simulink library "xpcmeasurementcomputinglib"  (Simulink 6.0)
settings: Solver=ode45  SolverMode=SingleTasking  StartTime=0.0  StopTime=10.0  RelTol=1e-3
values from neighbouring files (symbols this model uses):
  channels = round(channels)    [mbwaudpmc.m]
undefined symbols (not defined in the file or in its folder): madcbciodas, madcbpcidas, madcbpcidas1600, mctr05checks, mdacbisa, mdacbpcidas, mdacbpcidas1600, mdacbpcidda0x12, mdiocbpcipdisox, menccbcioquadcount, misa8255, mpci8255, mtccb
libraries: xpcmeasurementcomputinglib x18
(part 1 of 4)
settings Model: Creator=adowd  LastModifiedBy=gweast
settings DataIOCC: SignalLoggingName=logsOut
settings OptimizationCC: BooleanDataType=off
settings DebuggingCC: CheckExecutionContextPreStartOutputMsg=on  CheckExecutionContextRuntimeOutputMsg=on  SolverPrmCheckMsg=none
settings HardwareCC: TargetUnknown=on
settings GRTTargetCC: UtilityFuncGeneration=Automatic  LifeSpan=inf
settings SFSimCC: SFSimApplyToAllLibs=on  SFSimBuildMode=Incremental

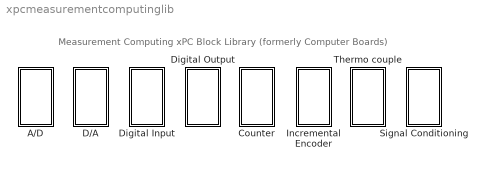
== system xpcmeasurementcomputinglib ==
  note: Measurement Computing xPC Block Library
      | (formerly Computer Boards)
  A/D : Subsystem  EnableExecutionContextPropagation=on
  Counter : Subsystem  EnableExecutionContextPropagation=on
  D/A : Subsystem  EnableExecutionContextPropagation=on
  Digital Input : Subsystem  EnableExecutionContextPropagation=on
  Digital Output : Subsystem  EnableExecutionContextPropagation=on
  Incremental Encoder : Subsystem  EnableExecutionContextPropagation=on
  Signal Conditioning : Subsystem  EnableExecutionContextPropagation=on
  Thermo couple : Subsystem  EnableExecutionContextPropagation=on

== system xpcmeasurementcomputinglib/A/D ==
  "CIO-DAS16 330 " : S-Function  InitFcn=madcbciodas(1);  FunctionName=adcbciodas  Parameters="channel, range, gain, offset, control, mux, sampletime, baseaddress,  boardType"  mask(adcbpcidas){channel=1, range=+-10V, mux=Single-ended (16 channels), sampletime=0.001, baseaddress=0x300}
      mask prompts: channel "Number of channels:"; range "Range vector:"; mux "Input coupling:"; sampletime "Sample time:"; baseaddress "Base address (i.e. 0xd000):"
      mask help:
      | CIO-DAS16/300
      | ComputerBoards
      | Analog Input
      mask init:
      | baseaddress=hex2dec(baseaddress(3:end));
      | boardType=4;gain=0;offset=0;control=0;
      | [gain, offset, control]=madcbciodas(2, channel, range, mux, baseaddress, boardType);
      mask Help: helpview(fullfile(docroot, 'mapfiles', 'xpc.map'), 'ComputerBoards_CIO-DAS16-330_AD')
      mask StyleString: edit,popup(+-10V|+-5V|+-2.5V|+-1.25V|+-0.625V|0-10V|0-5V|0-2.5V|0-1.25V),popup(Single-ended (16 channels)|differential (8 channels)),edit,edit
      mask Display: disp('CIO-DAS16/330\nComputerBoards\nAnalog Input');port_label('output',1,'1');
  "CIO-DAS16 JR " : S-Function  InitFcn=madcbciodas(1);  FunctionName=adcbciodas  Parameters="channel, range, gain, offset, control, mux, sampletime, baseaddress,  boardType"  mask(adcbpcidas){channel=1, range=+-10V, mux=Single-ended (16 channels), sampletime=0.001, baseaddress=0x300}
      mask prompts: channel "Number of channels:"; range "Range vector:"; mux "Input coupling:"; sampletime "Sample time:"; baseaddress "Base address (i.e. 0xd000):"
      mask help:
      | CIO-DAS16/JR
      | ComputerBoards
      | Analog Input
      mask init:
      | baseaddress=hex2dec(baseaddress(3:end));
      | boardType=1;gain=0;offset=0;control=0;
      | [gain, offset, control]=madcbciodas(2, channel, range, mux, baseaddress, boardType);
      mask Help: helpview(fullfile(docroot, 'mapfiles', 'xpc.map'), 'ComputerBoards_CIO-DAS16-JR_AD')
      mask StyleString: edit,popup(+-10V|+-5V|+-2.5V|+-1.25V|+-0.625V|0-10V|0-5V|0-2.5V|0-1.25V),popup(Single-ended (16 channels)|differential (8 channels)),edit,edit
      mask Display: disp('CIO-DAS16/JR\nComputerBoards\nAnalog Input');port_label('output',1,'1');
  "CIO-DAS1601 12 " : S-Function  InitFcn=madcbciodas(1);  FunctionName=adcbciodas  Parameters="channel, range, gain, offset, control, mux, sampletime, baseaddress,  boardType"  mask(adcbpcidas){channel=1, range=+-10V, mux=Single-ended (16 channels), sampletime=0.001, baseaddress=0x300}
      mask prompts: channel "Number of channels:"; range "Range vector:"; mux "Input coupling:"; sampletime "Sample time:"; baseaddress "Base address (i.e. 0xd000):"
      mask help:
      | CIO-DAS1601/12
      | ComputerBoards
      | Analog Input
      mask init:
      | baseaddress=hex2dec(baseaddress(3:end));
      | boardType=2;gain=0;offset=0;control=0;
      | [gain, offset, control]=madcbciodas(2, channel, range, mux, baseaddress, boardType);
      mask Help: helpview(fullfile(docroot, 'mapfiles', 'xpc.map'), 'ComputerBoards_CIO-DAS1601-12_AD')
      mask StyleString: edit,popup(+-10V|+-1V|+-0.1V|+-0.01V|0-10V|0-1V|0-0.1V|0-0.01V),popup(Single-ended (16 channels)|Differential (8 channels)),edit,edit
      mask Display: disp('CIO-DAS1601/12\nComputerBoards\nAnalog Input');port_label('output',1,'1');
  "CIO-DAS1602 12 " : S-Function  InitFcn=madcbciodas(1);  FunctionName=adcbciodas  Parameters="channel, range, gain, offset, control, mux, sampletime, baseaddress,  boardType"  mask(adcbpcidas){channel=1, range=+-10V, mux=Single-ended (16 channels), sampletime=0.001, baseaddress=0x300}
      mask prompts: channel "Number of channels:"; range "Range vector:"; mux "Input coupling:"; sampletime "Sample time:"; baseaddress "Base address (i.e. 0xd000):"
      mask help:
      | CIO-DAS1602/12
      | ComputerBoards
      | Analog Input
      mask init:
      | baseaddress=hex2dec(baseaddress(3:end));
      | boardType=3;gain=0;offset=0;control=0;
      | [gain, offset, control]=madcbciodas(2, channel, range, mux, baseaddress, boardType);
      mask Help: helpview(fullfile(docroot, 'mapfiles', 'xpc.map'), 'ComputerBoards_CIO-DAS1602-12_AD')
      mask StyleString: edit,popup(+-10V|+-5V|+-2.5V|+-1.25V|0-10V|0-5V|0-2.5V|0-1.25V),popup(Single-ended (16 channels)|Differential (8 channels)),edit,edit
      mask Display: disp('CIO-DAS1602/12\nComputerBoards\nAnalog Input');port_label('output',1,'1');
  "CIO-DAS1602 16 " : S-Function  InitFcn=madcbciodas(1);  FunctionName=adcbciodas  Parameters="channel, range, gain, offset, control, mux, sampletime, baseaddress,  boardType"  mask(adcbpcidas){channel=1, range=+-10V, mux=Single-ended (16 channels), sampletime=0.001, baseaddress=0x300}
      mask prompts: channel "Number of channels:"; range "Range vector:"; mux "Input coupling:"; sampletime "Sample time:"; baseaddress "Base address (i.e. 0xd000):"
      mask help:
      | CIO-DAS1602/16
      | ComputerBoards
      | Analog Input
      mask init:
      | baseaddress=hex2dec(baseaddress(3:end));
      | boardType=7;gain=0;offset=0;control=0;
      | [gain, offset, control]=madcbciodas(2, channel, range, mux, baseaddress, boardType);
      mask Help: helpview(fullfile(docroot, 'mapfiles', 'xpc.map'), 'ComputerBoards_CIO-DAS1602-16_AD')
      mask StyleString: edit,popup(+-10V|+-5V|+-2.5V|+-1.25V|+-0.625V|0-10V|0-5V|0-2.5V|0-1.25V),popup(Single-ended (16 channels)|differential (8 channels)),edit,edit
      mask Display: disp('CIO-DAS1602/16\nComputerBoards\nAnalog Input');port_label('output',1,'1');
  "CIO-DAS16JR 16 " : S-Function  InitFcn=madcbciodas(1);  FunctionName=adcbciodas  Parameters="channel, range, gain, offset, control, mux, sampletime, baseaddress,  boardType"  mask(adcbpcidas){channel=1, range=+-10V, mux=Single-ended (16 channels), sampletime=0.001, baseaddress=0x300}
      mask prompts: channel "Number of channels:"; range "Range vector:"; mux "Input coupling:"; sampletime "Sample time:"; baseaddress "Base address (i.e. 0xd000):"
      mask help:
      | CIO-DAS16JR/16
      | ComputerBoards
      | Analog Input
      mask init:
      | baseaddress=hex2dec(baseaddress(3:end));
      | boardType=6;gain=0;offset=0;control=0;
      | [gain, offset, control]=madcbciodas(2, channel, range, mux, baseaddress, boardType);
      mask Help: helpview(fullfile(docroot, 'mapfiles', 'xpc.map'), 'ComputerBoards_CIO-DAS16JR-16_AD')
      mask StyleString: edit,popup(+-10V|+-5V|+-2.5V|+-1.25V|+-0.625V|0-10V|0-5V|0-2.5V|0-1.25V),popup(Single-ended (16 channels)|differential (8 channels)),edit,edit
      mask Display: disp('CIO-DAS16JR/16\nComputerBoards\nAnalog Input');port_label('output',1,'1');
  "CIO-DAS16JR EXP " : Subsystem  EnableExecutionContextPropagation=on  mask(Analog Input Module){channels=[], gain=[], admux=0, range=+-10V, sampletime=0.001, baseaddress=0x300}
      mask prompts: channels "EXP channel vector:"; gain "EXP gain vector:"; admux "A/D board channel:"; range "A/D board range:"; sampletime "Sample time:"; baseaddress "Base address (i.e. 0xd000):"
      mask help:
      | Computer Boards
      | CIO-DAS16/Jr with EXP
      | Analog Input
      mask init:
      | baseaddress=hex2dec(baseaddress(3:end));
      mask Help: helpview(fullfile(docroot, 'mapfiles', 'xpc.map'), 'ComputerBoards_CIO-DAS16JR-EXP_AD')
      mask StyleString: edit,edit,popup(0|1|2|3|4|5|6|7|8|9|10|11|12|13|14|15),popup(+-10V|+-5V|+-2.5V|+-1.25V|+-0.625V|0-10V|0-5V|0-2.5V|0-1.25V),edit,edit
      mask Display: disp('CIO-DAS16/Jr EXP\nComputerBoards\nAnalog Input')
  "PC104-DAS16JR 12 " : S-Function  InitFcn=madcbciodas(1);  FunctionName=adcbciodas  Parameters="channel, range, gain, offset, control, mux, sampletime, baseaddress,  boardType"  mask(adcbpcidas){channel=1, range=+-10V, mux=Single-ended (16 channels), sampletime=0.001, baseaddress=0x300}
      mask prompts: channel "Number of channels:"; range "Range vector:"; mux "Input coupling:"; sampletime "Sample time:"; baseaddress "Base address (i.e. 0xd000):"
      mask help:
      | PC104-DAS16JR/12
      | ComputerBoards
      | Analog Input
      mask init:
      | baseaddress=hex2dec(baseaddress(3:end));
      | boardType=5;gain=0;offset=0;control=0;
      | [gain, offset, control]=madcbciodas(2, channel, range, mux, baseaddress, boardType);
      mask Help: helpview(fullfile(docroot, 'mapfiles', 'xpc.map'), 'ComputerBoards_PC104-DAS16JR-12_AD')
      mask StyleString: edit,popup(+-10V|+-5V|+-2.5V|+-1.25V|+-0.625V|0-10V|0-5V|0-2.5V|0-1.25V),popup(Single-ended (16 channels)|differential (8 channels)),edit,edit
      mask Display: disp('PC104-DAS16JR/12\nComputerBoards\nAnalog Input');port_label('output',1,'1');
  "PC104-DAS16JR 16 " : S-Function  InitFcn=madcbciodas(1);  FunctionName=adcbciodas  Parameters="channel, range, gain, offset, control, mux, sampletime, baseaddress,  boardType"  mask(adcbpcidas){channel=1, range=+-10V, mux=Single-ended (16 channels), sampletime=0.001, baseaddress=0x300}
      mask prompts: channel "Number of channels:"; range "Range vector:"; mux "Input coupling:"; sampletime "Sample time:"; baseaddress "Base address (i.e. 0xd000):"
      mask help:
      | PC104-DAS16JR/16
      | ComputerBoards
      | Analog Input
      mask init:
      | baseaddress=hex2dec(baseaddress(3:end));
      | boardType=8;gain=0;offset=0;control=0;
      | [gain, offset, control]=madcbciodas(2, channel, range, mux, baseaddress, boardType);
      mask Help: helpview(fullfile(docroot, 'mapfiles', 'xpc.map'), 'ComputerBoards_PC104-DAS16JR-16_AD')
      mask StyleString: edit,popup(+-10V|+-5V|+-2.5V|+-1.25V|+-0.625V|0-10V|0-5V|0-2.5V|0-1.25V),popup(Single-ended (16 channels)|differential (8 channels)),edit,edit
      mask Display: disp('PC104-DAS16JR/16\nComputerBoards\nAnalog Input');port_label('output',1,'1');
  "PCI-DAS1200 " : S-Function  InitFcn=madcbpcidas(1);  FunctionName=adcbpcidas  Parameters="channel, range, gain, offset, control, mux, sampletime, slot,  boardType"  mask(adcbpcidas){channel=1, range=+-10V, mux=Single-ended (16 channels), sampletime=0.001, slot=-1}
      mask prompts: channel "Number of channels:"; range "Range vector:"; mux "Input coupling:"; sampletime "Sample time:"; slot "PCI slot (-1: autosearch):"
      mask help:
      | PCI-DAS1200
      | ComputerBoards
      | Analog Input
      mask init:
      | boardType=1;gain=0;offset=0;control=0;
      | [gain, offset, control]=madcbpcidas(2, channel, range, mux, slot, boardType);
      mask Help: helpview(fullfile(docroot, 'mapfiles', 'xpc.map'), 'ComputerBoards_PCI-DAS1200_AD')
      mask StyleString: edit,popup(+-10V|+-5V|+-2.5V|+-1.25V|0-10V|0-5V|0-2.5V|0-1.25V),popup(Single-ended (16 channels)|Differential (8 channels)),edit,edit
      mask Display: disp('PCI-DAS1200\nComputerBoards\nAnalog Input');port_label('output',1,'1');
  "PCI-DAS1200 JR " : S-Function  InitFcn=madcbpcidas(1);  FunctionName=adcbpcidas  Parameters="channel, range, gain, offset, control, mux, sampletime, slot,  boardType"  mask(adcbpcidas){channel=1, range=+-10V, mux=Single-ended (16 channels), sampletime=0.001, slot=-1}
      mask prompts: channel "Number of channels:"; range "Range vector:"; mux "Input coupling:"; sampletime "Sample time:"; slot "PCI slot (-1: autosearch):"
      mask help:
      | PCI-DAS1200/JR
      | ComputerBoards
      | Analog Input
      mask init:
      | boardType=2;gain=0;offset=0;control=0;
      | [gain, offset, control]=madcbpcidas(2, channel, range, mux, slot, boardType);
      mask Help: helpview(fullfile(docroot, 'mapfiles', 'xpc.map'), 'ComputerBoards_PCI-DAS1200-JR_AD')
      mask StyleString: edit,popup(+-10V|+-5V|+-2.5V|+-1.25V|0-10V|0-5V|0-2.5V|0-1.25V),popup(Single-ended (16 channels)|Differential (8 channels)),edit,edit
      mask Display: disp('PCI-DAS1200/JR\nComputerBoards\nAnalog Input');port_label('output',1,'1');
  "PCI-DAS1602 12 " : S-Function  InitFcn=madcbpcidas1600(1);  FunctionName=adcbpcidas1600  Parameters="channel, range, gain, offset, control, mux, sampletime, slot,  boardType"  mask(adcbpcidas160212){channel=1, range=+-10V, mux=Single-ended (16 channels), sampletime=0.001, slot=-1}
      mask prompts: channel "Number of channels:"; range "Range vector:"; mux "Input coupling:"; sampletime "Sample time:"; slot "PCI slot (-1: autosearch):"
      mask help:
      | PCI-DAS1602/12
      | ComputerBoards
      | Analog Input
      mask init:
      | boardType=1;
      | control=0;
      | gain=0;
      | offset=0;
      | [gain, offset, control]=madcbpcidas1600(2, channel, range, mux, slot, boardType);
      mask Help: helpview(fullfile(docroot, 'mapfiles', 'xpc.map'), 'ComputerBoards_PCI-DAS1602-12_AD')
      mask StyleString: edit,popup(+-10V|+-5V|+-2.5V|+-1.25V|0-10V|0-5V|0-2.5V|0-1.25V),popup(Single-ended (16 channels)|Differential (8 channels)),edit,edit
      mask Display: disp('PCI-DAS1602/12\nComputerBoards\nAnalog Input');port_label('output',1,'1');
  "PCI-DAS1602 16 " : S-Function  InitFcn=madcbpcidas1600(1);  FunctionName=adcbpcidas1600  Parameters="channel, range, gain, offset, control, mux, sampletime, slot,  boardType"  mask(adcbpcidas160216){channel=1, range=+-10V, mux=Single-ended (16 channels), sampletime=0.001, slot=-1}
      mask prompts: channel "Number of channels:"; range "Range vector:"; mux "Input coupling:"; sampletime "Sample time:"; slot "PCI slot (-1: autosearch):"
      mask help:
      | PCI-DAS1602/16
      | ComputerBoards
      | Analog Input
      mask init:
      | boardType=2;
      | control=0;
      | gain=0;
      | offset=0;
      | [gain, offset, control]=madcbpcidas1600(2, channel, range, mux, slot, boardType);
      mask Help: helpview(fullfile(docroot, 'mapfiles', 'xpc.map'), 'ComputerBoards_PCI-DAS1602-16_AD')
      mask StyleString: edit,popup(+-10V|+-5V|+-2.5V|+-1.25V|0-10V|0-5V|0-2.5V|0-1.25V),popup(Single-ended (16 channels)|Differential (8 channels)),edit,edit
      mask Display: disp('PCI-DAS1602/16\nComputerBoards\nAnalog Input');port_label('output',1,'1');
  "PCIM-DAS1602 16 " : S-Function  InitFcn=madcbpcidas1600(1);  FunctionName=adcbpcidas1600  Parameters="channel, range, gain, offset, control, mux, sampletime, slot,  boardType"  mask(adcbpcimdas160216){channel=1, range=+-10V, mux=Single-ended (16 channels), sampletime=0.001, slot=-1}
      mask prompts: channel "Number of channels:"; range "Range vector:"; mux "Input coupling:"; sampletime "Sample time:"; slot "PCI slot (-1: autosearch):"
      mask help:
      | PCIM-DAS1602/16
      | ComputerBoards
      | Analog Input
      mask init:
      | boardType=3;
      | control=0;
      | gain=0;
      | offset=0;
      | [gain, offset, control]=madcbpcidas1600(2, channel, range, mux, slot, boardType);
      mask Help: helpview(fullfile(docroot, 'mapfiles', 'xpc.map'), 'ComputerBoards_PCIM-DAS1602-16_AD')
      mask StyleString: edit,popup(+-10V|+-5V|+-2.5V|+-1.25V|0-10V|0-5V|0-2.5V|0-1.25V),popup(Single-ended (16 channels)|Differential (8 channels)),edit,edit
      mask Display: disp('PCIM-DAS1602/16\nComputerBoards\nAnalog Input');port_label('output',1,'1');

== system xpcmeasurementcomputinglib/Counter ==
  "CIO-CTR05 " : Subsystem  EnableExecutionContextPropagation=on  mask(PWM){counterin=1, freq_base=F1=1MHz, freq=0.001, seq=High - Low, level=High, Ts=0.001, baseAddress=0x300}
      mask prompts: counterin "Counter:"; freq_base "Frequency base:"; freq "Relative output frequency:"; seq "Level sequence of square wave:"; level "Level when disarmed:"; Ts "Sample time:"; baseAddress "Base address (i.e. 0xd000):"
      mask help:
      | CIO-CTR05
      | ComputerBoards
      | PWM
      mask init:
      | init_arm=0;
      | initduty=0.5;
      | counter=counterin;
      | if counter>5
      | counter=counter-5;
      | baseAddress=['0x',dec2hex(hex2dec(baseAddress(3:end))+4)];
      | end;
      | [MasterMode, CounterMode, Init, Runtime, Term] =pwmarm_amd9513(counter, freq_base, freq, initduty, level, init_arm);
      | level=level-1;
      | seq=seq-1;
      mask Help: helpview(fullfile(docroot, 'mapfiles', 'xpc.map'), 'ComputerBoards_CIO-CTR05_Counter')
      mask StyleString: popup(1|2|3|4|5),popup(F1=1MHz|F2=100KHz|F3=10kHz|F4=1kHz|F5=100Hz),edit,popup(High - Low|Low- High),popup(Low|High),edit,edit
      mask Display: text(0.95,0.75,'CIO-CTR05','horizontalAlignment','right');text(0.95,0.50,'ComputerBoards','horizontalAlignment','right');text(0.95,0.25,'PWM','horizontalAlignment','right');port_label('input',1,[num2str(counterin),' (dc)'] );
  CIO-CTR05 1 : Subsystem  EnableExecutionContextPropagation=on  mask(PWM){counterin=1, freq_base=F1=1MHz, freq=0.001, seq=High - Low, level=High, Ts=0.001, baseAddress=0x300}
      mask prompts: counterin "Counter:"; freq_base "Frequency base:"; freq "Relative output frequency:"; seq "Level sequence of square wave:"; level "Level when disarmed:"; Ts "Sample time:"; baseAddress "Base address (i.e. 0xd000):"
      mask help:
      | CIO-CTR05
      | ComputerBoards
      | PWM & ARM
      mask init: same as xpcmeasurementcomputinglib/Counter/CIO-CTR05 
      mask Help: helpview(fullfile(docroot, 'mapfiles', 'xpc.map'), 'ComputerBoards_CIO-CTR05-1_Counter')
      mask StyleString: popup(1|2|3|4|5),popup(F1=1MHz|F2=100KHz|F3=10kHz|F4=1kHz|F5=100Hz),edit,popup(High - Low|Low- High),popup(Low|High),edit,edit
      mask Display: text(0.95,0.75,'CIO-CTR05','horizontalAlignment','right');text(0.95,0.50,'ComputerBoards','horizontalAlignment','right');text(0.95,0.25,'PWM & ARM','horizontalAlignment','right');port_label('input',1,[num2str(counterin),' (dc)'] );port_label('input',2,[num2str(counterin),' (arm)'] );
  CIO-CTR05 2 : Subsystem  EnableExecutionContextPropagation=on  mask(PWM){counterin=1, freq_base=F1=1MHz, duty=0.001, seq=High - Low, level=High, Ts=0.001, baseAddress=0x300}
      mask prompts: counterin "Counter:"; freq_base "Frequency base:"; duty "Output duty cycle:"; seq "Level sequence of square wave:"; level "Level when disarmed:"; Ts "Sample time:"; baseAddress "Base address (i.e. 0xd000):"
      mask help:
      | CIO-CTR05
      | ComputerBoards
      | FM
      mask init:
      | init_arm=0;
      | initfreq=0.005;
      | counter=counterin;
      | if counter>5
      | counter=counter-5;
      | baseAddress=['0x',dec2hex(hex2dec(baseAddress(3:end))+4)];
      | end;
      | [MasterMode, CounterMode, Init, Runtime, Term] =fmarm_amd9513(counter, freq_base, duty, initfreq, level, init_arm);
      | level=level-1;
      | seq=seq-1;
      mask Help: helpview(fullfile(docroot, 'mapfiles', 'xpc.map'), 'ComputerBoards_CIO-CTR05-2_Counter')
      mask StyleString: popup(1|2|3|4|5),popup(F1=1MHz|F2=100KHz|F3=10kHz|F4=1kHz|F5=100Hz),edit,popup(High - Low|Low- High),popup(Low|High),edit,edit
      mask Display: text(0.95,0.75,'CIO-CTR05','horizontalAlignment','right');text(0.95,0.50,'ComputerBoards','horizontalAlignment','right');text(0.95,0.25,'FM','horizontalAlignment','right');port_label('input',1,[num2str(counterin),' (f)'] );
  CIO-CTR05 3 : Subsystem  EnableExecutionContextPropagation=on  mask(FM){counterin=1, freq_base=F1=1MHz, duty=0.001, seq=High - Low, level=High, Ts=0.001, baseAddress=0x300}
      mask prompts: counterin "Counter:"; freq_base "Frequency base:"; duty "Output duty cycle:"; seq "Level sequence of square wave:"; level "Level when disarmed:"; Ts "Sample time:"; baseAddress "Base address (i.e. 0xd000):"
      mask help:
      | CIO-CTR05
      | ComputerBoards
      | FM & ARM
      mask init: same as xpcmeasurementcomputinglib/Counter/CIO-CTR05 2
      mask Help: helpview(fullfile(docroot, 'mapfiles', 'xpc.map'), 'ComputerBoards_CIO-CTR05-3_Counter')
      mask StyleString: popup(1|2|3|4|5),popup(F1=1MHz|F2=100KHz|F3=10kHz|F4=1kHz|F5=100Hz),edit,popup(High - Low|Low- High),popup(Low|High),edit,edit
      mask Display: text(0.95,0.75,'CIO-CTR05','horizontalAlignment','right');text(0.95,0.50,'ComputerBoards','horizontalAlignment','right');text(0.95,0.25,'FM & ARM','horizontalAlignment','right');port_label('input',1,[num2str(counterin),' (f)'] );port_label('input',2,[num2str(counterin),' (arm)'] );
  CIO-CTR05 4 : Subsystem  EnableExecutionContextPropagation=on  mask(PWMcap){counterin=1&2, freq_base=F1=1MHz, Ts=0.001, baseAddress=0x300}
      mask prompts: counterin "Counter:"; freq_base "Frequency base:"; Ts "Sample time:"; baseAddress "Base address (i.e. 0xd000):"
      mask help:
      | CIO-CTR05
      | ComputerBoards
      | PWM capture
      mask init:
      | counter=counterin;
      | if counter>4
      | counter=counter-4;
      | baseAddress=['0x',dec2hex(hex2dec(baseAddress(3:end))+4)];
      | end;
      | [MasterMode, CounterMode, Init, Runtime, Term] =pwmcap_amd9513(counter, freq_base);
      mask Help: helpview(fullfile(docroot, 'mapfiles', 'xpc.map'), 'ComputerBoards_CIO-CTR05-4_Counter')
      mask StyleString: popup(1&2|2&3|3&4|4&5),popup(F1=1MHz|F2=100KHz|F3=10kHz|F4=1kHz|F5=100Hz),edit,edit
      mask Display: text(0.05,0.75,'CIO-CTR05','horizontalAlignment','left');text(0.05,0.50,'ComputerBoards','horizontalAlignment','left');text(0.05,0.25,'PWM capture','horizontalAlignment','left');port_label('output',1,[num2str(counterin),' (f)'] );port_label('output',2,[num2str(counterin+1),' (dc)'] );
  CIO-CTR05 5 : Subsystem  EnableExecutionContextPropagation=on  mask(FREQcap){counterin=1, freq_base=F1=1MHz, Ts=0.001, baseAddress=0x300}
      mask prompts: counterin "Counter:"; freq_base "Frequency base:"; Ts "Sample time:"; baseAddress "Base address (i.e. 0xd000):"
      mask help:
      | CIO-CTR05
      | ComputerBoards
      | Frequency capture
      mask init:
      | counter=counterin;
      | if counter>5
      | counter=counter-5;
      | baseAddress=['0x',dec2hex(hex2dec(baseAddress(3:end))+4)];
      | end;
      | [MasterMode, CounterMode, Init, Runtime, Term] =freqcap_amd9513(counter, freq_base);
      mask Help: helpview(fullfile(docroot, 'mapfiles', 'xpc.map'), 'ComputerBoards_CIO-CTR05-5_Counter')
      mask StyleString: popup(1|2|3|4|5),popup(F1=1MHz|F2=100KHz|F3=10kHz|F4=1kHz|F5=100Hz),edit,edit
      mask Display: text(0.05,0.75,'CIO-CTR05','horizontalAlignment','left');text(0.05,0.50,'ComputerBoards','horizontalAlignment','left');text(0.05,0.25,'Freq. capture','horizontalAlignment','left');port_label('output',1,[num2str(counterin),' (f)'] );
  "CIO-CTR10 " : Subsystem  EnableExecutionContextPropagation=on  mask(PWM){counterin=1, freq_base=F1=1MHz, freq=0.001, seq=High - Low, level=High, Ts=0.001, baseAddress=0x300}
      mask prompts: counterin "Counter:"; freq_base "Frequency base:"; freq "Relative output frequency:"; seq "Level sequence of square wave:"; level "Level when disarmed:"; Ts "Sample time:"; baseAddress "Base address (i.e. 0xd000):"
      mask help:
      | CIO-CTR10
      | ComputerBoards
      | PWM
      mask init: same as xpcmeasurementcomputinglib/Counter/CIO-CTR05 
      mask Help: helpview(fullfile(docroot, 'mapfiles', 'xpc.map'), 'ComputerBoards_CIO-CTR10_Counter')
      mask StyleString: popup(1|2|3|4|5|6|7|8|9|10),popup(F1=1MHz|F2=100KHz|F3=10kHz|F4=1kHz|F5=100Hz),edit,popup(High - Low|Low- High),popup(Low|High),edit,edit
      mask Display: text(0.95,0.75,'CIO-CTR10','horizontalAlignment','right');text(0.95,0.50,'ComputerBoards','horizontalAlignment','right');text(0.95,0.25,'PWM','horizontalAlignment','right');port_label('input',1,[num2str(counterin),' (dc)'] );
  CIO-CTR10 1 : Subsystem  EnableExecutionContextPropagation=on  mask(PWM){counterin=1, freq_base=F1=1MHz, freq=0.001, seq=High - Low, level=High, Ts=0.001, baseAddress=0x300}
      mask prompts: counterin "Counter:"; freq_base "Frequency base:"; freq "Relative output frequency:"; seq "Level sequence of square wave:"; level "Level when disarmed:"; Ts "Sample time:"; baseAddress "Base address (i.e. 0xd000):"
      mask help:
      | CIO-CTR10
      | ComputerBoards
      | PWM & ARM
      mask init: same as xpcmeasurementcomputinglib/Counter/CIO-CTR05 
      mask Help: helpview(fullfile(docroot, 'mapfiles', 'xpc.map'), 'ComputerBoards_CIO-CTR10-1_Counter')
      mask StyleString: popup(1|2|3|4|5|6|7|8|9|10),popup(F1=1MHz|F2=100KHz|F3=10kHz|F4=1kHz|F5=100Hz),edit,popup(High - Low|Low- High),popup(Low|High),edit,edit
      mask Display: text(0.95,0.75,'CIO-CTR10','horizontalAlignment','right');text(0.95,0.50,'ComputerBoards','horizontalAlignment','right');text(0.95,0.25,'PWM & ARM','horizontalAlignment','right');port_label('input',1,[num2str(counterin),' (dc)'] );port_label('input',2,[num2str(counterin),' (arm)'] );
  CIO-CTR10 2 : Subsystem  EnableExecutionContextPropagation=on  mask(PWM){counterin=1, freq_base=F1=1MHz, duty=0.001, seq=High - Low, level=High, Ts=0.001, baseAddress=0x300}
      mask prompts: counterin "Counter:"; freq_base "Frequency base:"; duty "Output duty cycle:"; seq "Level sequence of square wave:"; level "Level when disarmed:"; Ts "Sample time:"; baseAddress "Base address (i.e. 0xd000):"
      mask help:
      | CIO-CTR10
      | ComputerBoards
      | FM
      mask init: same as xpcmeasurementcomputinglib/Counter/CIO-CTR05 2
      mask Help: helpview(fullfile(docroot, 'mapfiles', 'xpc.map'), 'ComputerBoards_CIO-CTR10-2_Counter')
      mask StyleString: popup(1|2|3|4|5|6|7|8|9|10),popup(F1=1MHz|F2=100KHz|F3=10kHz|F4=1kHz|F5=100Hz),edit,popup(High - Low|Low- High),popup(Low|High),edit,edit
      mask Display: text(0.95,0.75,'CIO-CTR10','horizontalAlignment','right');text(0.95,0.50,'ComputerBoards','horizontalAlignment','right');text(0.95,0.25,'FM','horizontalAlignment','right');port_label('input',1,[num2str(counterin),' (f)'] );
  CIO-CTR10 3 : Subsystem  EnableExecutionContextPropagation=on  mask(FM){counterin=1, freq_base=F1=1MHz, duty=0.001, seq=High - Low, level=High, Ts=0.001, baseAddress=0x300}
      mask prompts: counterin "Counter:"; freq_base "Frequency base:"; duty "Output duty cycle:"; seq "Level sequence of square wave:"; level "Level when disarmed:"; Ts "Sample time:"; baseAddress "Base address (i.e. 0xd000):"
      mask help:
      | CIO-CTR10
      | ComputerBoards
      | FM & ARM
      mask init: same as xpcmeasurementcomputinglib/Counter/CIO-CTR05 2
      mask Help: helpview(fullfile(docroot, 'mapfiles', 'xpc.map'), 'ComputerBoards_CIO-CTR10-3_Counter')
      mask StyleString: popup(1|2|3|4|5|6|7|8|9|10),popup(F1=1MHz|F2=100KHz|F3=10kHz|F4=1kHz|F5=100Hz),edit,popup(High - Low|Low- High),popup(Low|High),edit,edit
      mask Display: text(0.95,0.75,'CIO-CTR10','horizontalAlignment','right');text(0.95,0.50,'ComputerBoards','horizontalAlignment','right');text(0.95,0.25,'FM & ARM','horizontalAlignment','right');port_label('input',1,[num2str(counterin),' (f)'] );port_label('input',2,[num2str(counterin),' (arm)'] );
  CIO-CTR10 4 : Subsystem  EnableExecutionContextPropagation=on  mask(PWMcap){counterin=1&2, freq_base=F1=1MHz, Ts=0.001, baseAddress=0x300}
      mask prompts: counterin "Counter:"; freq_base "Frequency base:"; Ts "Sample time:"; baseAddress "Base address (i.e. 0xd000):"
      mask help:
      | CIO-CTR10
      | ComputerBoards
      | PWM capture
      mask init:
      | counter=counterin;
      | if counter>4
      | counter=counter-4;
      | baseAddress=['0x',dec2hex(hex2dec(baseAddress(3:end))+4)];
      | end;
      | [MasterMode, CounterMode, Init, Runtime, Term] =pwmcap_amd9513(counter, freq_base);
      mask Help: helpview(fullfile(docroot, 'mapfiles', 'xpc.map'), 'ComputerBoards_CIO-CTR10-4_Counter')
      mask StyleString: popup(1&2|2&3|3&4|4&5|6&7|7&8|8&9|9&10),popup(F1=1MHz|F2=100KHz|F3=10kHz|F4=1kHz|F5=100Hz),edit,edit
      mask Display: text(0.05,0.75,'CIO-CTR10','horizontalAlignment','left');text(0.05,0.50,'ComputerBoards','horizontalAlignment','left');text(0.05,0.25,'PWM capture','horizontalAlignment','left');port_label('output',1,[num2str(counterin),' (f)'] );port_label('output',2,[num2str(counterin+1),' (dc)'] );
  CIO-CTR10 5 : Subsystem  EnableExecutionContextPropagation=on  mask(FREQcap){counterin=1, freq_base=F1=1MHz, Ts=0.001, baseAddress=0x300}
      mask prompts: counterin "Counter:"; freq_base "Frequency base:"; Ts "Sample time:"; baseAddress "Base address (i.e. 0xd000):"
      mask help:
      | CIO-CTR10
      | ComputerBoards
      | Frequency capture
      mask init:
      | counter=counterin;
      | if counter>5
      | counter=counter-5;
      | baseAddress=['0x',dec2hex(hex2dec(baseAddress(3:end))+4)];
      | end;
      | [MasterMode, CounterMode, Init, Runtime, Term] =freqcap_amd9513(counter, freq_base);
      mask Help: helpview(fullfile(docroot, 'mapfiles', 'xpc.map'), 'ComputerBoards_CIO-CTR10-5_Counter')
      mask StyleString: popup(1|2|3|4|5|6|7|8|9|10),popup(F1=1MHz|F2=100KHz|F3=10kHz|F4=1kHz|F5=100Hz),edit,edit
      mask Display: text(0.05,0.75,'CIO-CTR10','horizontalAlignment','left');text(0.05,0.50,'ComputerBoards','horizontalAlignment','left');text(0.05,0.25,'Freq. capture','horizontalAlignment','left');port_label('output',1,[num2str(counterin),' (f)'] );
  "CIO-CTRxx " : S-Function  FunctionName=ctramd9513isa  Parameters=io, mm, cms, initir, ir, termir, ts, baseAddress  mask(cioctrxx){mastermode=[], countermode=[], init=[], commands=[], term=[], ts=0.001, baseAddress='0x300'}
      mask prompts: mastermode "Master mode structure:"; countermode "Counter mode structure:"; init "Initialization command structure:"; commands "Runtime command structure:"; term "Termination command structure:"; ts "Sample time:"; baseAddress "9513 chip base address (i.e. 0xd000):"
      mask help:
      | CIO-CTRxx
      | ComputerBoards
      | AMD9513 Counter
      mask init:
      | baseAddress=hex2dec(baseAddress(3:end));
      | [io,mm, cms, initir, ir, termir]=mamd9513parse(mastermode, countermode, init, commands, term);
      mask Help: helpview(fullfile(docroot, 'mapfiles', 'xpc.map'), 'ComputerBoards_CIO-CTRxx_Counter')
      mask Display: disp('AMD9513\nCounter')
  "PCI-CTR05 " : Subsystem  InitFcn=mctr05checks(1);  EnableExecutionContextPropagation=on  mask(PWM){counterin=1, freq_base=F1=5MHz, freq=0.01, seq=high - low, level=Low, Ts=0.001, pciSlot=-1}
      mask prompts: counterin "Counter:"; freq_base "Frequency base:"; freq "Relative output frequency:"; seq "Level sequence of square wave:"; level "Level when disarmed:"; Ts "Sample time:"; pciSlot "PCI slot (-1: autosearch):"
      mask help:
      | PCI-CTR05
      | ComputerBoards
      | PWM & ARM
      mask init:
      | init_arm=0;
      | initduty=0.5;
      | counter=counterin;
      | if counter>5
      | counter=counter-5;
      | end;
      | [MasterMode, CounterMode, Init, Runtime, Term] =pwmarm_amd9513(counter, freq_base, freq, initduty, level, init_arm);
      | level=level-1;
      | seq=seq-1;
      mask Help: helpview(fullfile(docroot, 'mapfiles', 'xpc.map'), 'ComputerBoards_PCI-CTR05_Counter')
      mask StyleString: popup(1|2|3|4|5),popup(F1=5MHz|F2=500KHz|F3=50kHz|F4=5kHz|F5=500Hz),edit,popup(high - low|low- high),popup(Low|High),edit,edit
      mask Display: text(0.95,0.75,'PCI-CTR05','horizontalAlignment','right');text(0.95,0.50,'ComputerBoards','horizontalAlignment','right');text(0.95,0.25,'PWM','horizontalAlignment','right');port_label('input',1,[num2str(counterin),' (dc)'] );
  "PCI-CTR05  " : S-Function  FunctionName=ctramd9513cbpcictr05  Parameters=io, mm, cms, initir, ir, termir, ts, pciSlot  mask(pcictr05){mastermode=[], countermode=[], init=[], commands=[], term=[], ts=0.001, pciSlot=-1}
      mask prompts: mastermode "Master mode structure:"; countermode "Counter mode structure:"; init "Initialization command structure:"; commands "Runtime command structure:"; term "Termination command structure:"; ts "Sample time:"; pciSlot "PCI slot (-1: autosearch):"
      mask help:
      | PCI-CTR05
      | ComputerBoards
      | AMD9513 Counter
      mask init:
      | [io,mm, cms, initir, ir, termir]=mamd9513parse(mastermode, countermode, init, commands, term);
      mask Help: helpview(fullfile(docroot, 'mapfiles', 'xpc.map'), 'ComputerBoards_PCI-CTR05_Counter')
      mask Display: disp('AMD9513\nCounter')
  PCI-CTR05 1 : Subsystem  InitFcn=mctr05checks(1);  EnableExecutionContextPropagation=on  mask(PWM){counterin=1, freq_base=F1=5MHz, freq=0.01, seq=high - low, level=Low, Ts=0.001, pciSlot=-1}
      mask prompts: counterin "Counter:"; freq_base "Frequency base:"; freq "Relative output frequency:"; seq "Level sequence of square wave:"; level "Level when disarmed:"; Ts "Sample time:"; pciSlot "PCI slot (-1: autosearch):"
      mask help:
      | PCI-CTR05
      | ComputerBoards
      | PWM & ARM
      mask init: same as xpcmeasurementcomputinglib/Counter/PCI-CTR05 
      mask Help: helpview(fullfile(docroot, 'mapfiles', 'xpc.map'), 'ComputerBoards_PCI-CTR05-1_Counter')
      mask StyleString: popup(1|2|3|4|5),popup(F1=5MHz|F2=500KHz|F3=50kHz|F4=5kHz|F5=500Hz),edit,popup(high - low|low- high),popup(Low|High),edit,edit
      mask Display: text(0.95,0.75,'PCI-CTR05','horizontalAlignment','right');text(0.95,0.50,'ComputerBoards','horizontalAlignment','right');text(0.95,0.25,'PWM & ARM','horizontalAlignment','right');port_label('input',1,[num2str(counterin),' (dc)'] );port_label('input',2,[num2str(counterin),' (arm)'] );
  PCI-CTR05 2 : Subsystem  InitFcn=mctr05checks(1);  EnableExecutionContextPropagation=on  mask(FM){counterin=1, freq_base=F1=5MHz, duty=0.5, seq=high - low, level=Low, Ts=0.001, pciSlot=-1}
      mask prompts: counterin "Counter:"; freq_base "Frequency base:"; duty "Output duty cycle:"; seq "Level sequence of square wave:"; level "Level when disarmed:"; Ts "Sample time:"; pciSlot "PCI slot (-1: autosearch):"
      mask help:
      | PCI-CTR05
      | ComputerBoards
      | FM
      mask init:
      | init_arm=0;
      | initfreq=0.005;
      | counter=counterin;
      | if counter>5
      | counter=counter-5;
      | end;
      | [MasterMode, CounterMode, Init, Runtime, Term] =fmarm_amd9513(counter, freq_base, duty, initfreq, level, init_arm);
      | level=level-1;
      | seq=seq-1;
      mask Help: helpview(fullfile(docroot, 'mapfiles', 'xpc.map'), 'ComputerBoards_PCI-CTR05-2_Counter')
      mask StyleString: popup(1|2|3|4|5),popup(F1=5MHz|F2=500KHz|F3=50kHz|F4=5kHz|F5=500Hz),edit,popup(high - low|low- high),popup(Low|High),edit,edit
      mask Display: text(0.95,0.75,'PCI-CTR05','horizontalAlignment','right');text(0.95,0.50,'ComputerBoards','horizontalAlignment','right');text(0.95,0.25,'FM','horizontalAlignment','right');port_label('input',1,[num2str(counterin),' (f)'] );
  PCI-CTR05 3 : Subsystem  InitFcn=mctr05checks(1);  EnableExecutionContextPropagation=on  mask(FM){counterin=1, freq_base=F1=5MHz, duty=0.5, seq=high - low, level=Low, Ts=0.001, pciSlot=-1}
      mask prompts: counterin "Counter:"; freq_base "Frequency base:"; duty "Output duty cycle:"; seq "Level sequence of square wave:"; level "Level when disarmed:"; Ts "Sample time:"; pciSlot "PCI slot (-1: autosearch):"
      mask help:
      | PCI-CTR05
      | ComputerBoards
      | FM & ARM
      mask init: same as xpcmeasurementcomputinglib/Counter/PCI-CTR05 2
      mask Help: helpview(fullfile(docroot, 'mapfiles', 'xpc.map'), 'ComputerBoards_PCI-CTR05-3_Counter')
      mask StyleString: popup(1|2|3|4|5),popup(F1=5MHz|F2=500KHz|F3=50kHz|F4=5kHz|F5=500Hz),edit,popup(high - low|low- high),popup(Low|High),edit,edit
      mask Display: text(0.95,0.75,'PCI-CTR05','horizontalAlignment','right');text(0.95,0.50,'ComputerBoards','horizontalAlignment','right');text(0.95,0.25,'FM & ARM','horizontalAlignment','right');port_label('input',1,[num2str(counterin),' (f)'] );port_label('input',2,[num2str(counterin),' (arm)'] );
  PCI-CTR05 4 : Subsystem  InitFcn=mctr05checks(1);  EnableExecutionContextPropagation=on  mask(PWMcap){counterin=1&2, freq_base=F1=5MHz, Ts=0.001, pciSlot=-1}
      mask prompts: counterin "Counter:"; freq_base "Frequency base:"; Ts "Sample time:"; pciSlot "PCI slot (-1: autosearch):"
      mask help:
      | PCI-CTR05
      | ComputerBoards
      | PWM capture
      mask init:
      | counter=counterin;
      | if counter>4
      | counter=counter-4;
      | end;
      | [MasterMode, CounterMode, Init, Runtime, Term] =pwmcap_amd9513(counter, freq_base);
      mask Help: helpview(fullfile(docroot, 'mapfiles', 'xpc.map'), 'ComputerBoards_PCI-CTR05-4_Counter')
      mask StyleString: popup(1&2|2&3|3&4|4&5),popup(F1=5MHz|F2=500KHz|F3=50kHz|F4=5kHz|F5=500Hz),edit,edit
      mask Display: text(0.05,0.75,'PCI-CTR05','horizontalAlignment','left');text(0.05,0.50,'ComputerBoards','horizontalAlignment','left');text(0.05,0.25,'PWM capture','horizontalAlignment','left');port_label('output',1,[num2str(counterin),' (f)'] );port_label('output',2,[num2str(counterin+1),' (dc)'] );
  PCI-CTR05 5 : Subsystem  InitFcn=mctr05checks(1);  EnableExecutionContextPropagation=on  mask(FREQcap){counterin=1, freq_base=F1=5MHz, Ts=0.001, pciSlot=-1}
      mask prompts: counterin "Counter:"; freq_base "Frequency base:"; Ts "Sample time:"; pciSlot "PCI slot (-1: autosearch):"
      mask help:
      | PCI-CTR05
      | ComputerBoards
      | Frequency capture
      mask init:
      | counter=counterin;
      | if counter>5
      | counter=counter-5;
      | end;
      | [MasterMode, CounterMode, Init, Runtime, Term] =freqcap_amd9513(counter, freq_base);
      mask Help: helpview(fullfile(docroot, 'mapfiles', 'xpc.map'), 'ComputerBoards_PCI-CTR05-5_Counter')
      mask StyleString: popup(1|2|3|4|5),popup(F1=5MHz|F2=500KHz|F3=50kHz|F4=5kHz|F5=500Hz),edit,edit
      mask Display: text(0.05,0.75,'PCI-CTR05','horizontalAlignment','left');text(0.05,0.50,'ComputerBoards','horizontalAlignment','left');text(0.05,0.25,'Freq. capture','horizontalAlignment','left');port_label('output',1,[num2str(counterin),' (f)'] );
